simulink model "ExperimentalLab1Assignments"  (R2020b)
settings: Solver=VariableStepAuto  StartTime=0.0  StopTime=10.0  RelTol=1e-3
undefined symbols (not defined in the file): Beq_hat, D_w, degs2rpm, gbox, J_eq, K, K_D, k_drv, K_I, K_P, Kw, mot, N_r, N_u, N_w, N_x, National_Instruments, PCIe, R_eq, rpm2rads, sens, stepAmplitude, T_L, tau_sf_hat
libraries: sldrtlib x9, simulink x1
settings Model: Creator=Musta  LastModifiedBy=Musta

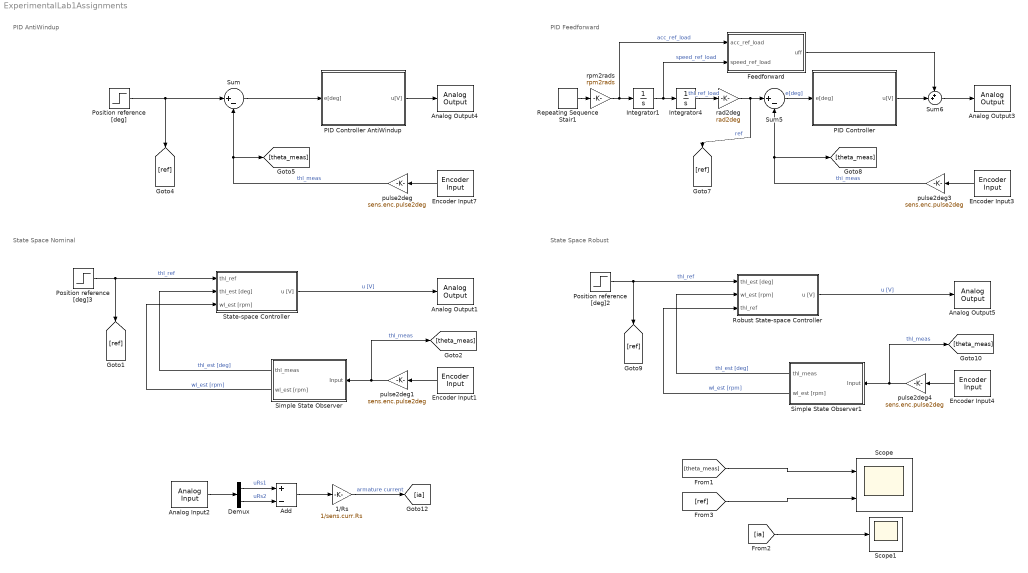
== system ExperimentalLab1Assignments ==
  note: PID AntiWindup
  note: State Space Nominal
  note: PID Feedforward
  note: State Space Robust
  1/Rs : Gain  Gain=1/sens.curr.Rs
  Add : Sum  Inputs=+-
  Analog Input2 : sldrtlib/Analog Input  SampleTime=0.001  MaxMissedTicks=10  ShowMissedTicks=off  YieldWhenWaiting=off  DrvName=National_Instruments/PCIe-6321  DrvAddress=4294967295  DrvOptions=[0 0 0 2 0 0 0]  Channels=[1,2]  RangeMode=1  VoltRange=1  DataType=1
      settings: AttributesFormatString=National Instruments\nPCIe-6321 [auto]
  Analog Output{1,3..5} (4 alike) : sldrtlib/Analog Output  SampleTime=0.001  MaxMissedTicks=10  ShowMissedTicks=off  YieldWhenWaiting=off  DrvName=National_Instruments/PCIe-6321  DrvAddress=4294967295  DrvOptions=[0 0 0 2 0 0 0]  Channels=1  RangeMode=1  VoltRange=1  InitialValue=0  FinalValue=0
      settings: AttributesFormatString=National Instruments\nPCIe-6321 [auto]
  Demux : Demux  Outputs=2
  Encoder Input{1,3..4,7} (4 alike) : sldrtlib/Encoder Input  SampleTime=0.001  MaxMissedTicks=10  ShowMissedTicks=off  YieldWhenWaiting=off  DrvName=National_Instruments/PCIe-6321  DrvAddress=4294967295  DrvOptions=[0 0 0 2 0 0 0]  Channels=1  QuadMode=3  IndexPulse=2  InputFilter=Inf  DataType=1
      settings: AttributesFormatString=National Instruments\nPCIe-6321 [auto]
  Feedforward : Subsystem
  Integrator1 : Integrator
  Integrator4 : Integrator
  PID Controller : Subsystem
  PID Controller AntiWindup : Subsystem
  Position reference [deg]2 : Step  Time=0  After=stepAmplitude  SampleTime=0
  Position reference [deg]3 : Step  Time=0  After=stepAmplitude  SampleTime=0
  Position reference [deg] : Step  After=stepAmplitude  SampleTime=0
  Repeating Sequence Stair1 : simulink/Sources/Repeating Sequence Stair  OutValues=[900 0 -900 -900 0 900]  tsamp=0.5  OutMin=[]  OutMax=[]  OutDataTypeStr=double  OutputDataTypeScalingMode=double  OutDataType=fixdt(0,8)  ConRadixGroup=Best Precision: Vector-wise  OutScaling=2^-12
  Robust State-space Controller : Subsystem
  Scope : Scope  NumInputPorts=2
  Scope1 : Scope
  Simple State Observer : Subsystem
  Simple State Observer1 : Subsystem
  State-space Controller : Subsystem
  Sum : Sum  Inputs=|+-
  Sum5 : Sum  Inputs=|+-
  Sum6 : Sum  Inputs=++|
  pulse2deg{,1,3..4} (4 alike) : Gain  Gain=sens.enc.pulse2deg
  rad2deg : Gain  Gain=rad2deg
  rpm2rads : Gain  Gain=rpm2rads
  wires:
  [ref] -> Scope/2
  PID Controller AntiWindup/1(u[V]) -> Analog Output4/1
  Position reference [deg]/1 -> Sum/1, [ref]
  [ia] -> Scope1/1
  Demux/1 -> Add/1  "uRs1"
  1/Rs/1 -> [ia]  "armature current"
  Encoder Input7/1 -> pulse2deg/1
  Analog Input2/1 -> Demux/1
  Add/1 -> 1/Rs/1
  Demux/2 -> Add/2  "uRs2"
  [theta_meas] -> Scope/1
  pulse2deg/1 -> [theta_meas], Sum/2  "thl_meas"
  Sum/1 -> PID Controller AntiWindup/1(e[deg])
  Encoder Input1/1 -> pulse2deg1/1
  pulse2deg1/1 -> [theta_meas], Simple State Observer/1(Input)  "thl_meas"
  Encoder Input3/1 -> pulse2deg3/1
  Sum6/1 -> Analog Output3/1
  Feedforward/1(uff) -> Sum6/1
  rad2deg/1 -> [ref], Sum5/1  "ref"
  rpm2rads/1 -> Feedforward/1(acc_ref_load), Integrator1/1  "acc_ref_load"
  Sum5/1 -> PID Controller/1(e[deg])  "e[deg]"
  Integrator1/1 -> Integrator4/1, Feedforward/2(speed_ref_load)  "speed_ref_load"
  Repeating Sequence Stair1/1 -> rpm2rads/1
  pulse2deg3/1 -> [theta_meas], Sum5/2  "thi_meas"
  Integrator4/1 -> rad2deg/1  "thl_ref_load"
  PID Controller/1(u[V]) -> Sum6/2
  State-space Controller/1(u [V]) -> Analog Output1/1  "u [V]"
  Simple State Observer/2(wl_est [rpm]) -> State-space Controller/3(wl_est [rpm])  "wl_est [rpm]"
  Simple State Observer/1(thl_meas) -> State-space Controller/2(thl_est [deg])  "thl_est [deg]"
  Position reference [deg]3/1 -> State-space Controller/1(thl_ref), [ref]  "thl_ref"
  Robust State-space Controller/1(u [V]) -> Analog Output5/1  "u [V]"
  Position reference [deg]2/1 -> Robust State-space Controller/1(thl_est [deg]), [ref]  "thl_ref"
  Simple State Observer1/2(wl_est [rpm]) -> Robust State-space Controller/3(thl_ref)  "wl_est [rpm]"
  pulse2deg4/1 -> Simple State Observer1/1(Input), [theta_meas]  "thl_meas"
  Encoder Input4/1 -> pulse2deg4/1
  Simple State Observer1/1(thl_meas) -> Robust State-space Controller/2(wl_est [rpm])  "thl_est [deg]"

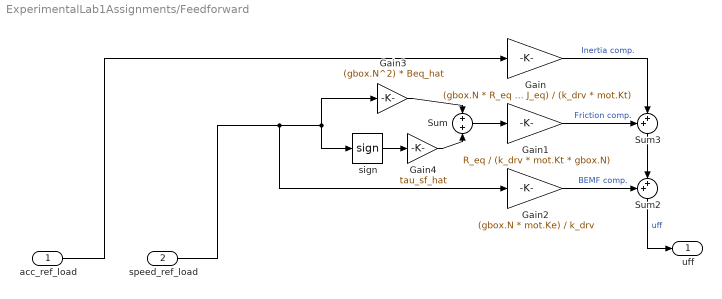
== system ExperimentalLab1Assignments/Feedforward ==
  acc_ref_load : Inport
  speed_ref_load : Inport  Port=2
  Gain : Gain  Gain=(gbox.N * R_eq * J_eq) / (k_drv * mot.Kt)
  Gain1 : Gain  Gain=R_eq / (k_drv * mot.Kt * gbox.N)
  Gain2 : Gain  Gain=(gbox.N * mot.Ke) / k_drv
  Gain3 : Gain  Gain=(gbox.N^2) * Beq_hat
  Gain4 : Gain  Gain=tau_sf_hat
  Sum : Sum  Inputs=+|+
  Sum2 : Sum  Inputs=++|
  Sum3 : Sum  Inputs=++|
  sign : Signum
  uff : Outport
  wires:
  sign/1 -> Gain4/1
  Sum/1 -> Gain1/1
  speed_ref_load/1 -> Gain2/1, sign/1, Gain3/1
  Sum3/1 -> Sum2/2
  Gain3/1 -> Sum/1
  Gain/1 -> Sum3/2  "Inertia comp."
  Gain1/1 -> Sum3/1  "Friction comp."
  Gain4/1 -> Sum/2
  Gain2/1 -> Sum2/1  "BEMF comp."
  acc_ref_load/1 -> Gain/1
  Sum2/1 -> uff/1  "uff"

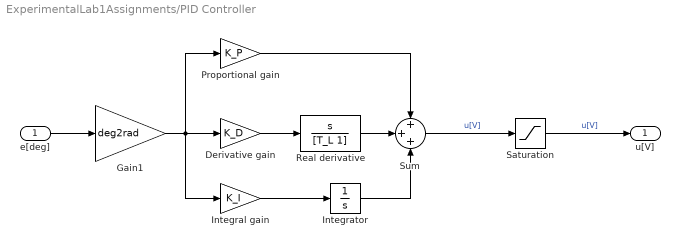
== system ExperimentalLab1Assignments/PID Controller ==
  e[deg] : Inport
  Derivative gain : Gain  Gain=K_D
  Gain1 : Gain  Gain=deg2rad
  Integral gain : Gain  Gain=K_I
  Integrator : Integrator
  Proportional gain : Gain  Gain=K_P
  Real derivative : TransferFcn  Numerator=[1 0]  Denominator=[T_L 1]
  Saturation : Saturate  UpperLimit=10  LowerLimit=-10
  Sum : Sum  Inputs=+++
  u[V] : Outport
  wires:
  e[deg]/1 -> Gain1/1
  Real derivative/1 -> Sum/2
  Gain1/1 -> Derivative gain/1, Integral gain/1, Proportional gain/1
  Proportional gain/1 -> Sum/1
  Integrator/1 -> Sum/3
  Derivative gain/1 -> Real derivative/1
  Sum/1 -> Saturation/1  "u[V]"
  Saturation/1 -> u[V]/1  "u[V]"
  Integral gain/1 -> Integrator/1

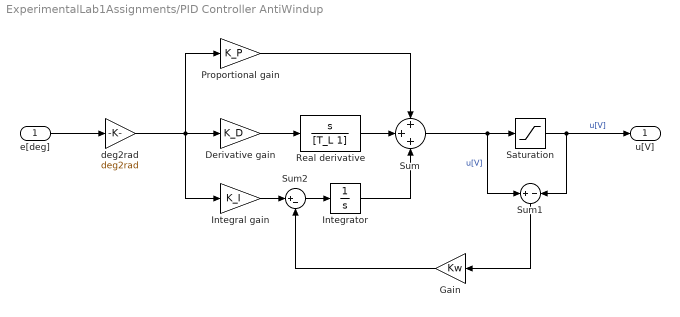
== system ExperimentalLab1Assignments/PID Controller AntiWindup ==
  e[deg] : Inport
  Derivative gain : Gain  Gain=K_D
  Gain : Gain  Gain=Kw
  Integral gain : Gain  Gain=K_I
  Integrator : Integrator
  Proportional gain : Gain  Gain=K_P
  Real derivative : TransferFcn  Numerator=[1 0]  Denominator=[T_L 1]
  Saturation : Saturate  UpperLimit=10  LowerLimit=-10
  Sum : Sum  Inputs=+++
  Sum1 : Sum  Inputs=+|-
  Sum2 : Sum  Inputs=|+-
  deg2rad : Gain  Gain=deg2rad
  u[V] : Outport
  wires:
  e[deg]/1 -> deg2rad/1
  Real derivative/1 -> Sum/2
  deg2rad/1 -> Proportional gain/1, Derivative gain/1, Integral gain/1
  Proportional gain/1 -> Sum/1
  Integrator/1 -> Sum/3
  Derivative gain/1 -> Real derivative/1
  Sum/1 -> Saturation/1, Sum1/1  "u[V]"
  Saturation/1 -> Sum1/2, u[V]/1  "u[V]"
  Sum1/1 -> Gain/1
  Integral gain/1 -> Sum2/1
  Sum2/1 -> Integrator/1
  Gain/1 -> Sum2/2

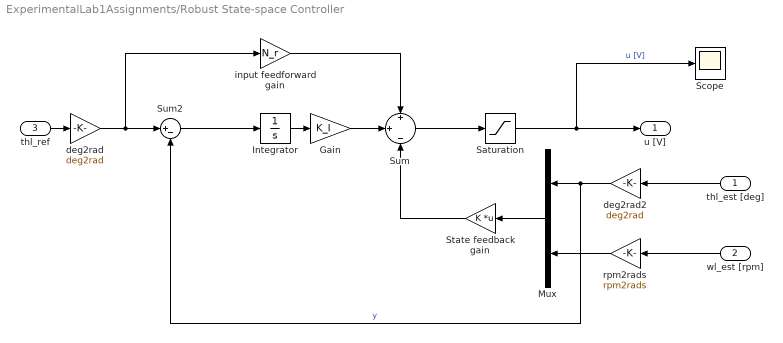
== system ExperimentalLab1Assignments/Robust State-space Controller ==
  thl_est [deg] : Inport
  wl_est [rpm] : Inport  Port=2
  thl_ref : Inport  Port=3
  Gain : Gain  Gain=K_I
  Integrator : Integrator
  Mux : Mux  Inputs=2
  Saturation : Saturate  UpperLimit=10  LowerLimit=-10
  Scope : Scope
  State feedback gain : Gain  Gain=K  Multiplication=Matrix(K*u)
  Sum : Sum  Inputs=+|+|-
  Sum2 : Sum  Inputs=|+-
  deg2rad : Gain  Gain=deg2rad
  deg2rad2 : Gain  Gain=deg2rad
  input feedforward gain : Gain  Gain=N_r
  rpm2rads : Gain  Gain=rpm2rads
  u [V] : Outport
  wires:
  input feedforward gain/1 -> Sum/1
  Mux/1 -> State feedback gain/1
  deg2rad/1 -> Sum2/1, input feedforward gain/1
  Saturation/1 -> u [V]/1, Scope/1  "u [V]"
  rpm2rads/1 -> Mux/2
  deg2rad2/1 -> Sum2/2, Mux/1  "y"
  Integrator/1 -> Gain/1
  Gain/1 -> Sum/2
  State feedback gain/1 -> Sum/3
  Sum/1 -> Saturation/1
  Sum2/1 -> Integrator/1
  thl_est [deg]/1 -> deg2rad2/1
  wl_est [rpm]/1 -> rpm2rads/1
  thl_ref/1 -> deg2rad/1

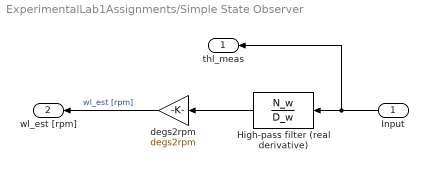
== system ExperimentalLab1Assignments/Simple State Observer ==
  Input : Inport
  High-pass filter (real derivative) : TransferFcn  Numerator=N_w  Denominator=D_w
  degs2rpm : Gain  Gain=degs2rpm
  thl_meas : Outport
  wl_est [rpm] : Outport  Port=2
  wires:
  Input/1 -> thl_meas/1, High-pass filter (real derivative)/1
  High-pass filter (real derivative)/1 -> degs2rpm/1
  degs2rpm/1 -> wl_est [rpm]/1  "wl_est [rpm]"

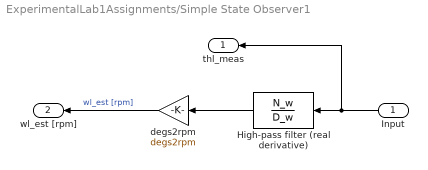
== system ExperimentalLab1Assignments/Simple State Observer1 ==
  Input : Inport
  High-pass filter (real derivative) : TransferFcn  Numerator=N_w  Denominator=D_w
  degs2rpm : Gain  Gain=degs2rpm
  thl_meas : Outport
  wl_est [rpm] : Outport  Port=2
  wires:
  Input/1 -> thl_meas/1, High-pass filter (real derivative)/1
  High-pass filter (real derivative)/1 -> degs2rpm/1
  degs2rpm/1 -> wl_est [rpm]/1  "wl_est [rpm]"

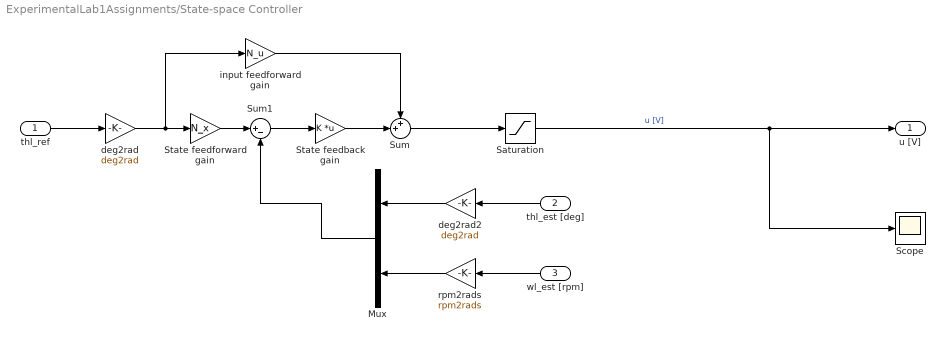
== system ExperimentalLab1Assignments/State-space Controller ==
  thl_ref : Inport
  thl_est [deg] : Inport  Port=2
  wl_est [rpm] : Inport  Port=3
  Mux : Mux  Inputs=2
  Saturation : Saturate  UpperLimit=10  LowerLimit=-10
  Scope : Scope
  State feedback gain : Gain  Gain=K  Multiplication=Matrix(K*u)
  State feedforward gain : Gain  Gain=N_x
  Sum : Sum  Inputs=++|
  Sum1 : Sum  Inputs=|+-
  deg2rad : Gain  Gain=deg2rad
  deg2rad2 : Gain  Gain=deg2rad
  input feedforward gain : Gain  Gain=N_u
  rpm2rads : Gain  Gain=rpm2rads
  u [V] : Outport
  wires:
  input feedforward gain/1 -> Sum/1
  Mux/1 -> Sum1/2
  State feedforward gain/1 -> Sum1/1
  State feedback gain/1 -> Sum/2
  deg2rad/1 -> input feedforward gain/1, State feedforward gain/1
  Sum1/1 -> State feedback gain/1
  Sum/1 -> Saturation/1
  thl_ref/1 -> deg2rad/1
  Saturation/1 -> Scope/1, u [V]/1  "u [V]"
  rpm2rads/1 -> Mux/2
  wl_est [rpm]/1 -> rpm2rads/1
  thl_est [deg]/1 -> deg2rad2/1
  deg2rad2/1 -> Mux/1
